simulink model "threelevel_12phase1"  (R2020b)
settings: Solver=FixedStepDiscrete  StartTime=0.0  StopTime=1  FixedStep=Ts_FEA  RelTol=1e-3
model workspace (MAT data in the model file):
  T_10kHz : Simulink.Parameter (value not decoded)
undefined symbols (not defined in the file): Cin, DiscIntNeverNeededParam, ESL, ESR, faif, Jm, kfeed_r, ki_n, kp_n, L, Ld, Line, Lq, ncmd_climb, ncmd_cruise, ncmd_run, ncmd_takeoff, p, Pcmd_climb, Pcmd_cruise, Pcmd_run, Pcmd_takeoff, Rs, Tcmd_run, Tcmd_start, Tcmd_time, time_climb, time_cruise, time_run, time_start, time_takeoff, Ts, Ts_Dead, Ts_FEA, Ts_speedloop, tswitch_climb, tswitch_takeoff, VDC, ws, zero_C1
libraries: powerlib x73, simulink x16, powerlib_meascontrol x16, slpidlib x13
(part 3 of 6)

== matlab function threelevel_12phase1/CurrentLoop/Subsystem/NTSV_7_nearest ==
  data: Alpha input; Beta input; Ta1 output; Ta2 output; Tb1 output; Tb2 output; Tc1 output; Tc2 output; r input; r output
function [Ta1,Ta2,Tb1, Tb2,Tc1,Tc2,r]  = fcn(Alpha,Beta,r)
temp1=Beta;
temp2=0.8660254*Alpha+Beta*0.5;
temp3=temp2-temp1;%0.8660254*Alpha-0.5beta
VecSector1=3;
VecSector2=1;
VecSector3=0;
if temp2>0
    VecSector1=VecSector1-1;
end
if temp3>0
    VecSector1=VecSector1-1;
end
if temp1<0
    VecSector1=7-VecSector1;
end 
switch VecSector1
    case {1,4}  
       if(abs(temp2)>0.5)
           VecSector2=VecSector2+1;
           if(abs(temp3)<0.5)
               VecSector2=VecSector2+1;
               if(abs(temp1)>0.5)
                   VecSector2=VecSector2+1;
               end
           end
       end
       if(temp1<temp3)
           VecSector3=1;
       else
           VecSector3=2;
       end
    case {2,5}
       if(abs(temp1)>0.5)
           VecSector2=VecSector2+1;
           if(abs(temp2)<0.5)
               VecSector2=VecSector2+1;
               if(abs(temp3)>0.5)
                   VecSector2=VecSector2+1;
               end
           end
       end
       if(temp2+temp3>0)
          VecSector3=1;
       else
           VecSector3=2;
       end 
    case {3,6}
       if(abs(temp3)>0.5)
           VecSector2=VecSector2+1;
           if(abs(temp1)<0.5)
               VecSector2=VecSector2+1;
               if(abs(temp2)>0.5)
                   VecSector2=VecSector2+1;
               end
           end
       end
       if(temp1+temp2>0)
          VecSector3=1;
       else
           VecSector3=2;
       end 
    otherwise
        VecSector1=0;
        VecSector2=0;
end
switch VecSector1
    case 1
        switch VecSector2
            case 1
                if(VecSector3==1)
                    Ta1=temp3;
                    Ta2=1;
                    Tb1=0;
                    Tb2=1-temp3;
                    Tc1=0;
                    Tc2=1-temp2-temp1;

                    Tb2=Tb2+Ta1*r;
                    Tc2=Tc2+Ta1*r;
                    Ta1=Ta1+Ta1*r;
                elseif(VecSector3==2)
                    Ta1=temp2+temp3;
                    Ta2=1;
                    Tb1=temp1;
                    Tb2=1;
                    Tc1=0;
                    Tc2=1-temp1;

                    Tc2=Tc2+Tb1*r;
                    Ta1=Ta1+Tb1*r;
                    Tb1=Tb1+Tb1*r;
                else
                    Ta1=temp3;
                    Ta2=1;
                    Tb1=0;
                    Tb2=1-temp3;
                    Tc1=0;
                    Tc2=1-temp2-temp1;

                    Tb2=Tb2+Ta1*r;
                    Tc2=Tc2+Ta1*r;
                    Ta1=Ta1+Ta1*r;
                end
            case 2
                Ta1=temp2;
                Ta2=1;
                Tb1=0;
                Tb2=1-temp3+temp1;
                Tc1=0;
                Tc2=1-temp2;
                
                Ta1=Ta1+Tc2*r;
                Tb2=Tb2+Tc2*r;
                Tc2=Tc2+Tc2*r;
            case 3
                if(VecSector3==1)
                    Ta1=temp2+temp3-0.5;
                    Ta2=1;
                    Tb1=0;
                    Tb2=0.5+temp1;
                    Tc1=0;
                    Tc2=0.5-temp1;

                    Ta1=Ta1+Tc2*r;
                    Tb2=Tb2+Tc2*r;
                    Tc2=Tc2+Tc2*r;
                elseif(VecSector3==2)
                    Ta1=0.5+temp3;
                    Ta2=1;
                    Tb1=0.5-temp3;
                    Tb2=1;
                    Tc1=0;
                    Tc2=1.5-temp1-temp2;

                    Ta1=Ta1+Tb1*r;
                    Tc2=Tc2+Tb1*r;
                    Tb1=Tb1+Tb1*r;
                else
                    Ta1=temp2+temp3-0.5;
                    Ta2=1;
                    Tb1=0;
                    Tb2=0.5+temp1;
                    Tc1=0;
                    Tc2=0.5-temp1;

                    Ta1=Ta1+Tc2*r;
                    Tb2=Tb2+Tc2*r;
                    Tc2=Tc2+Tc2*r;
                end
            case 4
                Ta1=temp2;
                Ta2=1;
                Tb1=temp1-temp3;
                Tb2=1;
                Tc1=0;
                Tc2=1-temp2;

                Ta1=Ta1+Tc2*r;
                Tb1=Tb1+Tc2*r;
                Tc2=Tc2+Tc2*r; 
            otherwise
                Ta1=0;
                Ta2=1;
                Tb1=0;
                Tb2=1;
                Tc1=0;
                Tc2=1;
        end
    case 2
        switch VecSector2
            case 1
                if(VecSector3==1)
                    Ta1=temp2;
                    Ta2=1;
                    Tb1=temp1-temp3;
                    Tb2=1;
                    Tc1=0;
                    Tc2=1-temp2;

                    Tb1=Tb1+Ta1*r;
                    Tc2=Tc2+Ta1*r;
                    Ta1=Ta1+Ta1*r;
                elseif(VecSector3==2)
                    Ta1=0;
                    Ta2=1+temp3;
                    Tb1=-temp3;
                    Tb2=1;
                    Tc1=0;
                    Tc2=1-temp2-temp1;
                    
                    Tc2=Tc2+Tb1*r;
                    Ta2=Ta2+Tb1*r;
                    Tb1=Tb1+Tb1*r;
                else
                    Ta1=temp2;
                    Ta2=1;
                    Tb1=temp1-temp3;
                    Tb2=1;
                    Tc1=0;
                    Tc2=1-temp2;

                    Tb1=Tb1+Ta1*r;
                    Tc2=Tc2+Ta1*r;
                    Ta1=Ta1+Ta1*r;
                end
            case 2
                Ta1=temp2+temp3;
                Ta2=1;
                Tb1=temp1;
                Tb2=1;
                Tc1=0;
                Tc2=1-temp1;
                
                Ta1=Ta1+Tc2*r;
                Tb1=Tb1+Tc2*r;
                Tc2=Tc2+Tc2*r;
            case 3
                if(VecSector3==1)
                    Ta1=0.5+temp3;
                    Ta2=1;
                    Tb1=0.5-temp3;
                    Tb2=1;
                    Tc1=0;
                    Tc2=1.5-temp2-temp1;

                    Tb1=Tb1+Ta1*r;
                    Tc2=Tc2+Ta1*r;
                    Ta1=Ta1+Ta1*r;
                elseif(VecSector3==2)
                    Ta1=0;
                    Ta2=0.5+temp2;
                    Tb1=temp1-temp3-0.5;
                    Tb2=1;
                    Tc1=0;
                    Tc2=0.5-temp2;

                    Tb1=Tb1+Tc2*r;
                    Ta2=Ta2+Tc2*r;
                    Tc2=Tc2+Tc2*r;
                else
                    Ta1=0.5+temp3;
                    Ta2=1;
                    Tb1=0.5-temp3;
                    Tb2=1;
                    Tc1=0;
                    Tc2=1.5-temp2-temp1;

                    Tb1=Tb1+Ta1*r;
                    Tc2=Tc2+Ta1*r;
                    Ta1=Ta1+Ta1*r;
                end
            case 4
                Ta1=0;
                Ta2=1+temp2+temp3;
                Tb1=temp1;
                Tb2=1;
                Tc1=0;
                Tc2=1-temp1;
                
                Ta2=Ta2+Tc2*r;
                Tb1=Tb1+Tc2*r;
                Tc2=Tc2+Tc2*r;
            otherwise
                Ta1=0;
                Ta2=1;
                Tb1=0;
                Tb2=1;
                Tc1=0;
                Tc2=1;
        end
    case 3
        switch VecSector2
            case 1
                if(VecSector3==1)
                    Ta1=0;
                    Ta2=1+temp2+temp3;
                    Tb1=temp1;
                    Tb2=1;
                    Tc1=0;
                    Tc2=1-temp1;

                    Ta2=Ta2+Tb1*r;
                    Tc2=Tc2+Tb1*r;
                    Tb1=Tb1+Tb1*r;
                elseif(VecSector3==2)
                    Ta1=0;
                    Ta2=1+temp2;
                    Tb1=temp1-temp3;
                    Tb2=1;
                    Tc1=-temp2;
                    Tc2=1;

                    Ta2=Ta2+Tc1*r;
                    Tb1=Tb1+Tc1*r;
                    Tc1=Tc1+Tc1*r;
                else
                    Ta1=0;
                    Ta2=1+temp2+temp3;
                    Tb1=temp1;
                    Tb2=1;
                    Tc1=0;
                    Tc2=1-temp1;

                    Ta2=Ta2+Tb1*r;
                    Tc2=Tc2+Tb1*r;
                    Tb1=Tb1+Tb1*r;
                end
            case 2
                Ta1=0;
                Ta2=1+temp3;
                Tb1=-temp3;
                Tb2=1;
                Tc1=0;
                Tc2=1-temp2-temp1;

                Tb1=Tb1+Ta2*r;
                Tc2=Tc2+Ta2*r;
                Ta2=Ta2+Ta2*r;
            case 3
                if(VecSector3==1)
                    Ta1=0;
                    Ta2=0.5+temp2;
                    Tb1=-0.5-temp3+temp1;
                    Tb2=1;
                    Tc1=0;
                    Tc2=0.5-temp2;

                    Tb1=Tb1+Ta2*r;
                    Tc2=Tc2+Ta2*r;
                    Ta2=Ta2+Ta2*r;
                elseif(VecSector3==2)
                    Ta1=0;
                    Ta2=1.5+temp2+temp3;
                    Tb1=0.5+temp1;
                    Tb2=1;
                    Tc1=0.5-temp1;
                    Tc2=1;

                    Tb1=Tb1+Tc1*r;
                    Ta2=Ta2+Tc1*r;
                    Tc1=Tc1+Tc1*r;
                else
                    Ta1=0;
                    Ta2=0.5+temp2;
                    Tb1=-0.5-temp3+temp1;
                    Tb2=1;
                    Tc1=0;
                    Tc2=0.5-temp2;

                    Tb1=Tb1+Ta2*r;
                    Tc2=Tc2+Ta2*r;
                    Ta2=Ta2+Ta2*r; 
                end
            case 4
                Ta1=0;
                Ta2=1+temp3;
                Tb1=-temp3;
                Tb2=1;
                Tc1=-temp2-temp1;
                Tc2=1;
                
                Tb1=Tb1+Ta2*r;
                Tc1=Tc1+Ta2*r;
                Ta2=Ta2+Ta2*r;
            otherwise
                Ta1=0;
                Ta2=1;
                Tb1=0;
                Tb2=1;
                Tc1=0;
                Tc2=1;
        end
    case 4
        switch VecSector2
            case 1
                if(VecSector3==2)
                    Ta1=0;
                    Ta2=1+temp3;
                    Tb1=-temp3;
                    Tb2=1;
                    Tc1=-temp2-temp1;
                    Tc2=1;

                    Ta2=Ta2+Tb1*r;
                    Tc1=Tc1+Tb1*r;
                    Tb1=Tb1+Tb1*r;
                elseif(VecSector3==1)
                    Ta1=0;
                    Ta2=1+temp3+temp2;
                    Tb1=0;
                    Tb2=1+temp1;
                    Tc1=-temp1;
                    Tc2=1;

                    Ta2=Ta2+Tc1*r;
                    Tb2=Tb2+Tc1*r;
                    Tc1=Tc1+Tc1*r;
                else
                    Ta1=0;
                    Ta2=1+temp3;
                    Tb1=-temp3;
                    Tb2=1;
                    Tc1=-temp2-temp1;
                    Tc2=1;

                    Ta2=Ta2+Tb1*r;
                    Tc1=Tc1+Tb1*r;
                    Tb1=Tb1+Tb1*r;
                end
            case 2
                Ta1=0;
                Ta2=1+temp2;
                Tb1=temp1-temp3;
                Tb2=1;
                Tc1=-temp2;
                Tc2=1;
                
                Tb1=Tb1+Ta2*r;
                Tc1=Tc1+Ta2*r;
                Ta2=Ta2+Ta2*r;
            case 3
                if(VecSector3==2)
                    Ta1=0;
                    Ta2=1.5+temp2+temp3;
                    Tb1=0.5+temp1;
                    Tb2=1;
                    Tc1=0.5-temp1;
                    Tc2=1;

                    Ta2=Ta2+Tb1*r;
                    Tc1=Tc1+Tb1*r;
                    Tb1=Tb1+Tb1*r;
                elseif(VecSector3==1)
                    Ta1=0;
                    Ta2=0.5+temp3;
                    Tb1=0;
                    Tb2=0.5-temp3;
                    Tc1=-0.5-temp2-temp1;
                    Tc2=1;

                    Tc1=Tc1+Ta2*r;
                    Tb2=Tb2+Ta2*r;
                    Ta2=Ta2+Ta2*r;
                else
                    Ta1=0;
                    Ta2=1.5+temp2+temp3;
                    Tb1=0.5+temp1;
                    Tb2=1;
                    Tc1=0.5-temp1;
                    Tc2=1;

                    Ta2=Ta2+Tb1*r;
                    Tc1=Tc1+Tb1*r;
                    Tb1=Tb1+Tb1*r;
                end
            case 4
                Ta1=0;
                Ta2=1+temp2;
                Tb1=0;
                Tb2=1+temp1-temp3;
                Tc1=-temp2;
                Tc2=1;
                
                Tc1=Tc1+Ta2*r;
                Tb2=Tb2+Ta2*r;
                Ta2=Ta2+Ta2*r;
            otherwise
                Ta1=0;
                Ta2=1;
                Tb1=0;
                Tb2=1;
                Tc1=0;
                Tc2=1;
        end
    case 5
        switch VecSector2
            case 1
                if(VecSector3==2)
                    Ta1=0;
                    Ta2=1+temp2;
                    Tb1=0;
                    Tb2=1-temp3+temp1;
                    Tc1=-temp2;
                    Tc2=1;

                    Ta2=Ta2+Tc1*r;
                    Tb2=Tb2+Tc1*r;
                    Tc1=Tc1+Tc1*r;
                elseif(VecSector3==1)
                    Ta1=temp3;
                    Ta2=1;
                    Tb1=0;
                    Tb2=1-temp3;
                    Tc1=-temp2-temp1;
                    Tc2=1;

                    Tb2=Tb2+Ta1*r;
                    Tc1=Tc1+Ta1*r;
                    Ta1=Ta1+Ta1*r;
                else
                    Ta1=0;
                    Ta2=1+temp2;
                    Tb1=0;
                    Tb2=1-temp3+temp1;
                    Tc1=-temp2;
                    Tc2=1;

                    Ta2=Ta2+Tc1*r;
                    Tb2=Tb2+Tc1*r;
                    Tc1=Tc1+Tc1*r; 
                end
            case 2
                Ta1=0;
                Ta2=1+temp2+temp3;
                Tb1=0;
                Tb2=1+temp1;
                Tc1=-temp1;
                Tc2=1;
                
                Ta2=Ta2+Tb2*r;
                Tc1=Tc1+Tb2*r;
                Tb2=Tb2+Tb2*r;
            case 3
                if(VecSector3==2)
                    Ta1=0;
                    Ta2=0.5+temp3;
                    Tb1=0;
                    Tb2=0.5-temp3;
                    Tc1=-0.5-temp1-temp2;
                    Tc2=1;

                    Ta2=Ta2+Tb2*r;
                    Tc1=Tc1+Tb2*r;
                    Tb2=Tb2+Tb2*r;
                elseif(VecSector3==1)
                    Ta1=0.5+temp2;
                    Ta2=1;
                    Tb1=0;
                    Tb2=1.5-temp3+temp1;
                    Tc1=0.5-temp2;
                    Tc2=1;
 
                    Tc1=Tc1+Ta1*r;
                    Tb2=Tb2+Ta1*r;
                    Ta1=Ta1+Ta1*r;
                else
                    Ta1=0;
                    Ta2=0.5+temp3;
                    Tb1=0;
                    Tb2=0.5-temp3;
                    Tc1=-0.5-temp1-temp2;
                    Tc2=1;

                    Ta2=Ta2+Tb2*r;
                    Tc1=Tc1+Tb2*r;
                    Tb2=Tb2+Tb2*r;
                end
            case 4
                Ta1=temp2+temp3;
                Ta2=1;
                Tb1=0;
                Tb2=1+temp1;
                Tc1=-temp1;
                Tc2=1;
                
                Ta1=Ta1+Tb2*r;
                Tc1=Tc1+Tb2*r;
                Tb2=Tb2+Tb2*r;
            otherwise
                Ta1=0;
                Ta2=1;
                Tb1=0;
                Tb2=1;
                Tc1=0;
                Tc2=1;
        end
    case 6
        switch VecSector2
            case 1
                if(VecSector3==2)
                    Ta1=temp2+temp3;
                    Ta2=1;
                    Tb1=0;
                    Tb2=1+temp1;
                    Tc1=-temp1;
                    Tc2=1;

                    Ta1=Ta1+Tc1*r;
                    Tb2=Tb2+Tc1*r;
                    Tc1=Tc1+Tc1*r;
                elseif(VecSector3==1)
                    Ta1=temp2;
                    Ta2=1;
                    Tb1=0;
                    Tb2=1+temp1-temp3;
                    Tc1=0;
                    Tc2=1-temp2;

                    Tb2=Tb2+Ta1*r;
                    Tc2=Tc2+Ta1*r;
                    Ta1=Ta1+Ta1*r;
                else
                    Ta1=temp2+temp3;
                    Ta2=1;
                    Tb1=0;
                    Tb2=1+temp1;
                    Tc1=-temp1;
                    Tc2=1;

                    Ta1=Ta1+Tc1*r;
                    Tb2=Tb2+Tc1*r;
                    Tc1=Tc1+Tc1*r;
                end
            case 2
                Ta1=temp3;
                Ta2=1;
                Tb1=0;
                Tb2=1-temp3;
                Tc1=-temp2-temp1;
                Tc2=1;
                
                Ta1=Ta1+Tb2*r;
                Tc1=Tc1+Tb2*r;
                Tb2=Tb2+Tb2*r;
            case 3
                if(VecSector3==2)
                    Ta1=0.5+temp2;
                    Ta2=1;
                    Tb1=0;
                    Tb2=1.5+temp1-temp3;
                    Tc1=0.5-temp2;
                    Tc2=1;

                    Ta1=Ta1+Tc1*r;
                    Tb2=Tb2+Tc1*r;
                    Tc1=Tc1+Tc1*r;
                elseif(VecSector3==1)
                    Ta1=-0.5+temp2+temp3;
                    Ta2=1;
                    Tb1=0;
                    Tb2=0.5+temp1;
                    Tc1=0;
                    Tc2=0.5-temp1;

                    Ta1=Ta1+Tb2*r;
                    Tc2=Tc2+Tb2*r;
                    Tb2=Tb2+Tb2*r;
                else
                    Ta1=0.5+temp2;
                    Ta2=1;
                    Tb1=0;
                    Tb2=1.5+temp1-temp3;
                    Tc1=0.5-temp2;
                    Tc2=1;

                    Ta1=Ta1+Tc1*r;
                    Tb2=Tb2+Tc1*r;
                    Tc1=Tc1+Tc1*r;
                end
            case 4
                Ta1=temp3;
                Ta2=1;
                Tb1=0;
                Tb2=1-temp3;
                Tc1=0;
                Tc2=1-temp2-temp1;
                
                Ta1=Ta1+Tb2*r;
                Tc2=Tc2+Tb2*r;
                Tb2=Tb2+Tb2*r;
            otherwise
                Ta1=0;
                Ta2=1;
                Tb1=0;
                Tb2=1;
                Tc1=0;
                Tc2=1;
        end
    otherwise
        Ta1=0;
        Ta2=1;
        Tb1=0;
        Tb2=1;
        Tc1=0;
        Tc2=1;
end

== matlab function threelevel_12phase1/CurrentLoop/Subsystem2/NTSV_7_nearest ==
  data: Alpha input; Beta input; Ta1 output; Ta2 output; Tb1 output; Tb2 output; Tc1 output; Tc2 output; r input; r output
function [Ta1,Ta2,Tb1, Tb2,Tc1,Tc2,r]  = fcn(Alpha,Beta,r)
temp1=Beta;
temp2=0.8660254*Alpha+Beta*0.5;
temp3=temp2-temp1;%0.8660254*Alpha-0.5beta
VecSector1=3;
VecSector2=1;
VecSector3=0;
if temp2>0
    VecSector1=VecSector1-1;
end
if temp3>0
    VecSector1=VecSector1-1;
end
if temp1<0
    VecSector1=7-VecSector1;
end 
switch VecSector1
    case {1,4}  
       if(abs(temp2)>0.5)
           VecSector2=VecSector2+1;
           if(abs(temp3)<0.5)
               VecSector2=VecSector2+1;
               if(abs(temp1)>0.5)
                   VecSector2=VecSector2+1;
               end
           end
       end
       if(temp1<temp3)
           VecSector3=1;
       else
           VecSector3=2;
       end
    case {2,5}
       if(abs(temp1)>0.5)
           VecSector2=VecSector2+1;
           if(abs(temp2)<0.5)
               VecSector2=VecSector2+1;
               if(abs(temp3)>0.5)
                   VecSector2=VecSector2+1;
               end
           end
       end
       if(temp2+temp3>0)
          VecSector3=1;
       else
           VecSector3=2;
       end 
    case {3,6}
       if(abs(temp3)>0.5)
           VecSector2=VecSector2+1;
           if(abs(temp1)<0.5)
               VecSector2=VecSector2+1;
               if(abs(temp2)>0.5)
                   VecSector2=VecSector2+1;
               end
           end
       end
       if(temp1+temp2>0)
          VecSector3=1;
       else
           VecSector3=2;
       end 
    otherwise
        VecSector1=0;
        VecSector2=0;
end
switch VecSector1
    case 1
        switch VecSector2
            case 1
                if(VecSector3==1)
                    Ta1=temp3;
                    Ta2=1;
                    Tb1=0;
                    Tb2=1-temp3;
                    Tc1=0;
                    Tc2=1-temp2-temp1;

                    Tb2=Tb2+Ta1*r;
                    Tc2=Tc2+Ta1*r;
                    Ta1=Ta1+Ta1*r;
                elseif(VecSector3==2)
                    Ta1=temp2+temp3;
                    Ta2=1;
                    Tb1=temp1;
                    Tb2=1;
                    Tc1=0;
                    Tc2=1-temp1;

                    Tc2=Tc2+Tb1*r;
                    Ta1=Ta1+Tb1*r;
                    Tb1=Tb1+Tb1*r;
                else
                    Ta1=temp3;
                    Ta2=1;
                    Tb1=0;
                    Tb2=1-temp3;
                    Tc1=0;
                    Tc2=1-temp2-temp1;

                    Tb2=Tb2+Ta1*r;
                    Tc2=Tc2+Ta1*r;
                    Ta1=Ta1+Ta1*r;
                end
            case 2
                Ta1=temp2;
                Ta2=1;
                Tb1=0;
                Tb2=1-temp3+temp1;
                Tc1=0;
                Tc2=1-temp2;
                
                Ta1=Ta1+Tc2*r;
                Tb2=Tb2+Tc2*r;
                Tc2=Tc2+Tc2*r;
            case 3
                if(VecSector3==1)
                    Ta1=temp2+temp3-0.5;
                    Ta2=1;
                    Tb1=0;
                    Tb2=0.5+temp1;
                    Tc1=0;
                    Tc2=0.5-temp1;

                    Ta1=Ta1+Tc2*r;
                    Tb2=Tb2+Tc2*r;
                    Tc2=Tc2+Tc2*r;
                elseif(VecSector3==2)
                    Ta1=0.5+temp3;
                    Ta2=1;
                    Tb1=0.5-temp3;
                    Tb2=1;
                    Tc1=0;
                    Tc2=1.5-temp1-temp2;

                    Ta1=Ta1+Tb1*r;
                    Tc2=Tc2+Tb1*r;
                    Tb1=Tb1+Tb1*r;
                else
                    Ta1=temp2+temp3-0.5;
                    Ta2=1;
                    Tb1=0;
                    Tb2=0.5+temp1;
                    Tc1=0;
                    Tc2=0.5-temp1;

                    Ta1=Ta1+Tc2*r;
                    Tb2=Tb2+Tc2*r;
                    Tc2=Tc2+Tc2*r;
                end
            case 4
                Ta1=temp2;
                Ta2=1;
                Tb1=temp1-temp3;
                Tb2=1;
                Tc1=0;
                Tc2=1-temp2;

                Ta1=Ta1+Tc2*r;
                Tb1=Tb1+Tc2*r;
                Tc2=Tc2+Tc2*r; 
            otherwise
                Ta1=0;
                Ta2=1;
                Tb1=0;
                Tb2=1;
                Tc1=0;
                Tc2=1;
        end
    case 2
        switch VecSector2
            case 1
                if(VecSector3==1)
                    Ta1=temp2;
                    Ta2=1;
                    Tb1=temp1-temp3;
                    Tb2=1;
                    Tc1=0;
                    Tc2=1-temp2;

                    Tb1=Tb1+Ta1*r;
                    Tc2=Tc2+Ta1*r;
                    Ta1=Ta1+Ta1*r;
                elseif(VecSector3==2)
                    Ta1=0;
                    Ta2=1+temp3;
                    Tb1=-temp3;
                    Tb2=1;
                    Tc1=0;
                    Tc2=1-temp2-temp1;
                    
                    Tc2=Tc2+Tb1*r;
                    Ta2=Ta2+Tb1*r;
                    Tb1=Tb1+Tb1*r;
                else
                    Ta1=temp2;
                    Ta2=1;
                    Tb1=temp1-temp3;
                    Tb2=1;
                    Tc1=0;
                    Tc2=1-temp2;

                    Tb1=Tb1+Ta1*r;
                    Tc2=Tc2+Ta1*r;
                    Ta1=Ta1+Ta1*r;
                end
            case 2
                Ta1=temp2+temp3;
                Ta2=1;
                Tb1=temp1;
                Tb2=1;
                Tc1=0;
                Tc2=1-temp1;
                
                Ta1=Ta1+Tc2*r;
                Tb1=Tb1+Tc2*r;
                Tc2=Tc2+Tc2*r;
            case 3
                if(VecSector3==1)
                    Ta1=0.5+temp3;
                    Ta2=1;
                    Tb1=0.5-temp3;
                    Tb2=1;
                    Tc1=0;
                    Tc2=1.5-temp2-temp1;

                    Tb1=Tb1+Ta1*r;
                    Tc2=Tc2+Ta1*r;
                    Ta1=Ta1+Ta1*r;
                elseif(VecSector3==2)
                    Ta1=0;
                    Ta2=0.5+temp2;
                    Tb1=temp1-temp3-0.5;
                    Tb2=1;
                    Tc1=0;
                    Tc2=0.5-temp2;

                    Tb1=Tb1+Tc2*r;
                    Ta2=Ta2+Tc2*r;
                    Tc2=Tc2+Tc2*r;
                else
                    Ta1=0.5+temp3;
                    Ta2=1;
                    Tb1=0.5-temp3;
                    Tb2=1;
                    Tc1=0;
                    Tc2=1.5-temp2-temp1;

                    Tb1=Tb1+Ta1*r;
                    Tc2=Tc2+Ta1*r;
                    Ta1=Ta1+Ta1*r;
                end
            case 4
                Ta1=0;
                Ta2=1+temp2+temp3;
                Tb1=temp1;
                Tb2=1;
                Tc1=0;
                Tc2=1-temp1;
                
                Ta2=Ta2+Tc2*r;
                Tb1=Tb1+Tc2*r;
                Tc2=Tc2+Tc2*r;
            otherwise
                Ta1=0;
                Ta2=1;
                Tb1=0;
                Tb2=1;
                Tc1=0;
                Tc2=1;
        end
    case 3
        switch VecSector2
            case 1
                if(VecSector3==1)
                    Ta1=0;
                    Ta2=1+temp2+temp3;
                    Tb1=temp1;
                    Tb2=1;
                    Tc1=0;
                    Tc2=1-temp1;

                    Ta2=Ta2+Tb1*r;
                    Tc2=Tc2+Tb1*r;
                    Tb1=Tb1+Tb1*r;
                elseif(VecSector3==2)
                    Ta1=0;
                    Ta2=1+temp2;
                    Tb1=temp1-temp3;
                    Tb2=1;
                    Tc1=-temp2;
                    Tc2=1;

                    Ta2=Ta2+Tc1*r;
                    Tb1=Tb1+Tc1*r;
                    Tc1=Tc1+Tc1*r;
                else
                    Ta1=0;
                    Ta2=1+temp2+temp3;
                    Tb1=temp1;
                    Tb2=1;
                    Tc1=0;
                    Tc2=1-temp1;

                    Ta2=Ta2+Tb1*r;
                    Tc2=Tc2+Tb1*r;
                    Tb1=Tb1+Tb1*r;
                end
            case 2
                Ta1=0;
                Ta2=1+temp3;
                Tb1=-temp3;
                Tb2=1;
                Tc1=0;
                Tc2=1-temp2-temp1;

                Tb1=Tb1+Ta2*r;
                Tc2=Tc2+Ta2*r;
                Ta2=Ta2+Ta2*r;
            case 3
                if(VecSector3==1)
                    Ta1=0;
                    Ta2=0.5+temp2;
                    Tb1=-0.5-temp3+temp1;
                    Tb2=1;
                    Tc1=0;
                    Tc2=0.5-temp2;

                    Tb1=Tb1+Ta2*r;
                    Tc2=Tc2+Ta2*r;
                    Ta2=Ta2+Ta2*r;
                elseif(VecSector3==2)
                    Ta1=0;
                    Ta2=1.5+temp2+temp3;
                    Tb1=0.5+temp1;
                    Tb2=1;
                    Tc1=0.5-temp1;
                    Tc2=1;

                    Tb1=Tb1+Tc1*r;
                    Ta2=Ta2+Tc1*r;
                    Tc1=Tc1+Tc1*r;
                else
                    Ta1=0;
                    Ta2=0.5+temp2;
                    Tb1=-0.5-temp3+temp1;
                    Tb2=1;
                    Tc1=0;
                    Tc2=0.5-temp2;

                    Tb1=Tb1+Ta2*r;
                    Tc2=Tc2+Ta2*r;
                    Ta2=Ta2+Ta2*r; 
                end
            case 4
                Ta1=0;
                Ta2=1+temp3;
                Tb1=-temp3;
                Tb2=1;
                Tc1=-temp2-temp1;
                Tc2=1;
                
                Tb1=Tb1+Ta2*r;
                Tc1=Tc1+Ta2*r;
                Ta2=Ta2+Ta2*r;
            otherwise
                Ta1=0;
                Ta2=1;
                Tb1=0;
                Tb2=1;
                Tc1=0;
                Tc2=1;
        end
    case 4
        switch VecSector2
            case 1
                if(VecSector3==2)
                    Ta1=0;
                    Ta2=1+temp3;
                    Tb1=-temp3;
                    Tb2=1;
                    Tc1=-temp2-temp1;
                    Tc2=1;

                    Ta2=Ta2+Tb1*r;
                    Tc1=Tc1+Tb1*r;
                    Tb1=Tb1+Tb1*r;
                elseif(VecSector3==1)
                    Ta1=0;
                    Ta2=1+temp3+temp2;
                    Tb1=0;
                    Tb2=1+temp1;
                    Tc1=-temp1;
                    Tc2=1;

                    Ta2=Ta2+Tc1*r;
                    Tb2=Tb2+Tc1*r;
                    Tc1=Tc1+Tc1*r;
                else
                    Ta1=0;
                    Ta2=1+temp3;
                    Tb1=-temp3;
                    Tb2=1;
                    Tc1=-temp2-temp1;
                    Tc2=1;

                    Ta2=Ta2+Tb1*r;
                    Tc1=Tc1+Tb1*r;
                    Tb1=Tb1+Tb1*r;
                end
            case 2
                Ta1=0;
                Ta2=1+temp2;
                Tb1=temp1-temp3;
                Tb2=1;
                Tc1=-temp2;
                Tc2=1;
                
                Tb1=Tb1+Ta2*r;
                Tc1=Tc1+Ta2*r;
                Ta2=Ta2+Ta2*r;
            case 3
                if(VecSector3==2)
                    Ta1=0;
                    Ta2=1.5+temp2+temp3;
                    Tb1=0.5+temp1;
                    Tb2=1;
                    Tc1=0.5-temp1;
                    Tc2=1;

                    Ta2=Ta2+Tb1*r;
                    Tc1=Tc1+Tb1*r;
                    Tb1=Tb1+Tb1*r;
                elseif(VecSector3==1)
                    Ta1=0;
                    Ta2=0.5+temp3;
                    Tb1=0;
                    Tb2=0.5-temp3;
                    Tc1=-0.5-temp2-temp1;
                    Tc2=1;

                    Tc1=Tc1+Ta2*r;
                    Tb2=Tb2+Ta2*r;
                    Ta2=Ta2+Ta2*r;
                else
                    Ta1=0;
                    Ta2=1.5+temp2+temp3;
                    Tb1=0.5+temp1;
                    Tb2=1;
                    Tc1=0.5-temp1;
                    Tc2=1;

                    Ta2=Ta2+Tb1*r;
                    Tc1=Tc1+Tb1*r;
                    Tb1=Tb1+Tb1*r;
                end
            case 4
                Ta1=0;
                Ta2=1+temp2;
                Tb1=0;
                Tb2=1+temp1-temp3;
                Tc1=-temp2;
                Tc2=1;
                
                Tc1=Tc1+Ta2*r;
                Tb2=Tb2+Ta2*r;
                Ta2=Ta2+Ta2*r;
            otherwise
                Ta1=0;
                Ta2=1;
                Tb1=0;
                Tb2=1;
                Tc1=0;
                Tc2=1;
        end
    case 5
        switch VecSector2
            case 1
                if(VecSector3==2)
                    Ta1=0;
                    Ta2=1+temp2;
                    Tb1=0;
                    Tb2=1-temp3+temp1;
                    Tc1=-temp2;
                    Tc2=1;

                    Ta2=Ta2+Tc1*r;
                    Tb2=Tb2+Tc1*r;
                    Tc1=Tc1+Tc1*r;
                elseif(VecSector3==1)
                    Ta1=temp3;
                    Ta2=1;
                    Tb1=0;
                    Tb2=1-temp3;
                    Tc1=-temp2-temp1;
                    Tc2=1;

                    Tb2=Tb2+Ta1*r;
                    Tc1=Tc1+Ta1*r;
                    Ta1=Ta1+Ta1*r;
                else
                    Ta1=0;
                    Ta2=1+temp2;
                    Tb1=0;
                    Tb2=1-temp3+temp1;
                    Tc1=-temp2;
                    Tc2=1;

                    Ta2=Ta2+Tc1*r;
                    Tb2=Tb2+Tc1*r;
                    Tc1=Tc1+Tc1*r; 
                end
            case 2
                Ta1=0;
                Ta2=1+temp2+temp3;
                Tb1=0;
                Tb2=1+temp1;
                Tc1=-temp1;
                Tc2=1;
                
                Ta2=Ta2+Tb2*r;
                Tc1=Tc1+Tb2*r;
                Tb2=Tb2+Tb2*r;
            case 3
                if(VecSector3==2)
                    Ta1=0;
                    Ta2=0.5+temp3;
                    Tb1=0;
                    Tb2=0.5-temp3;
                    Tc1=-0.5-temp1-temp2;
                    Tc2=1;

                    Ta2=Ta2+Tb2*r;
                    Tc1=Tc1+Tb2*r;
                    Tb2=Tb2+Tb2*r;
                elseif(VecSector3==1)
                    Ta1=0.5+temp2;
                    Ta2=1;
                    Tb1=0;
                    Tb2=1.5-temp3+temp1;
                    Tc1=0.5-temp2;
                    Tc2=1;
 
                    Tc1=Tc1+Ta1*r;
                    Tb2=Tb2+Ta1*r;
                    Ta1=Ta1+Ta1*r;
                else
                    Ta1=0;
                    Ta2=0.5+temp3;
                    Tb1=0;
                    Tb2=0.5-temp3;
                    Tc1=-0.5-temp1-temp2;
                    Tc2=1;

                    Ta2=Ta2+Tb2*r;
                    Tc1=Tc1+Tb2*r;
                    Tb2=Tb2+Tb2*r;
                end
            case 4
                Ta1=temp2+temp3;
                Ta2=1;
                Tb1=0;
                Tb2=1+temp1;
                Tc1=-temp1;
                Tc2=1;
                
                Ta1=Ta1+Tb2*r;
                Tc1=Tc1+Tb2*r;
                Tb2=Tb2+Tb2*r;
            otherwise
                Ta1=0;
                Ta2=1;
                Tb1=0;
                Tb2=1;
                Tc1=0;
                Tc2=1;
        end
    case 6
        switch VecSector2
            case 1
                if(VecSector3==2)
                    Ta1=temp2+temp3;
                    Ta2=1;
                    Tb1=0;
                    Tb2=1+temp1;
                    Tc1=-temp1;
                    Tc2=1;

                    Ta1=Ta1+Tc1*r;
                    Tb2=Tb2+Tc1*r;
                    Tc1=Tc1+Tc1*r;
                elseif(VecSector3==1)
                    Ta1=temp2;
                    Ta2=1;
                    Tb1=0;
                    Tb2=1+temp1-temp3;
                    Tc1=0;
                    Tc2=1-temp2;

                    Tb2=Tb2+Ta1*r;
                    Tc2=Tc2+Ta1*r;
                    Ta1=Ta1+Ta1*r;
                else
                    Ta1=temp2+temp3;
                    Ta2=1;
                    Tb1=0;
                    Tb2=1+temp1;
                    Tc1=-temp1;
                    Tc2=1;

                    Ta1=Ta1+Tc1*r;
                    Tb2=Tb2+Tc1*r;
                    Tc1=Tc1+Tc1*r;
                end
            case 2
                Ta1=temp3;
                Ta2=1;
                Tb1=0;
                Tb2=1-temp3;
                Tc1=-temp2-temp1;
                Tc2=1;
                
                Ta1=Ta1+Tb2*r;
                Tc1=Tc1+Tb2*r;
                Tb2=Tb2+Tb2*r;
            case 3
                if(VecSector3==2)
                    Ta1=0.5+temp2;
                    Ta2=1;
                    Tb1=0;
                    Tb2=1.5+temp1-temp3;
                    Tc1=0.5-temp2;
                    Tc2=1;

                    Ta1=Ta1+Tc1*r;
                    Tb2=Tb2+Tc1*r;
                    Tc1=Tc1+Tc1*r;
                elseif(VecSector3==1)
                    Ta1=-0.5+temp2+temp3;
                    Ta2=1;
                    Tb1=0;
                    Tb2=0.5+temp1;
                    Tc1=0;
                    Tc2=0.5-temp1;

                    Ta1=Ta1+Tb2*r;
                    Tc2=Tc2+Tb2*r;
                    Tb2=Tb2+Tb2*r;
                else
                    Ta1=0.5+temp2;
                    Ta2=1;
                    Tb1=0;
                    Tb2=1.5+temp1-temp3;
                    Tc1=0.5-temp2;
                    Tc2=1;

                    Ta1=Ta1+Tc1*r;
                    Tb2=Tb2+Tc1*r;
                    Tc1=Tc1+Tc1*r;
                end
            case 4
                Ta1=temp3;
                Ta2=1;
                Tb1=0;
                Tb2=1-temp3;
                Tc1=0;
                Tc2=1-temp2-temp1;
                
                Ta1=Ta1+Tb2*r;
                Tc2=Tc2+Tb2*r;
                Tb2=Tb2+Tb2*r;
            otherwise
                Ta1=0;
                Ta2=1;
                Tb1=0;
                Tb2=1;
                Tc1=0;
                Tc2=1;
        end
    otherwise
        Ta1=0;
        Ta2=1;
        Tb1=0;
        Tb2=1;
        Tc1=0;
        Tc2=1;
end

== matlab function threelevel_12phase1/CurrentLoop/NTSV_7_normol ==
  data: Alpha input; Beta input; Ta1 output; Ta2 output; Tb1 output; Tb2 output; Tc1 output; Tc2 output; r input; VecSector1 output
function [Ta1,Ta2,Tb1,Tb2,Tc1,Tc2,VecSector1]  = fcn(Alpha,Beta,r)
temp1=Beta;
temp2=0.8660254*Alpha+Beta*0.5;
temp3=temp2-temp1;%0.8660254*Alpha-0.5beta
VecSector1=3;
VecSector2=1;

if temp2>0
    VecSector1=VecSector1-1;
end
if temp3>0
    VecSector1=VecSector1-1;
end
if temp1<0
    VecSector1=7-VecSector1;
end 
switch VecSector1
    case {1,4}  
       if(abs(temp2)>0.5)
           VecSector2=VecSector2+1;
           if(abs(temp3)<0.5)
               VecSector2=VecSector2+1;
               if(abs(temp1)>0.5)
                   VecSector2=VecSector2+1;
               end
           end
       end
    case {2,5}
       if(abs(temp1)>0.5)
           VecSector2=VecSector2+1;
           if(abs(temp2)<0.5)
               VecSector2=VecSector2+1;
               if(abs(temp3)>0.5)
                   VecSector2=VecSector2+1;
               end
           end
       end
    case {3,6}
       if(abs(temp3)>0.5)
           VecSector2=VecSector2+1;
           if(abs(temp1)<0.5)
               VecSector2=VecSector2+1;
               if(abs(temp2)>0.5)
                   VecSector2=VecSector2+1;
               end
           end
       end
    otherwise
        VecSector1=0;
        VecSector2=0;
end

switch VecSector1
    case 1
        switch VecSector2
            case 1
                Ta1=temp3;
                Ta2=1;
                Tb1=0;
                Tb2=1-temp3;
                Tc1=0;
                Tc2=1-temp2-temp1;

                Tb2=Tb2+Ta1*r;
                Tc2=Tc2+Ta1*r;
                Ta1=Ta1+Ta1*r;
            case 2
                Ta1=temp2;
                Ta2=1;
                Tb1=0;
                Tb2=1-temp3+temp1;
                Tc1=0;
                Tc2=1-temp2;
                
                Ta1=Ta1+Tc2*r;
                Tb2=Tb2+Tc2*r;
                Tc2=Tc2+Tc2*r;
            case 3
                Ta1=temp2+temp3-0.5;
                Ta2=1;
                Tb1=0;
                Tb2=0.5+temp1;
                Tc1=0;
                Tc2=0.5-temp1;

                Ta1=Ta1+Tc2*r;
                Tb2=Tb2+Tc2*r;
                Tc2=Tc2+Tc2*r;
            case 4
                Ta1=temp2;
                Ta2=1;
                Tb1=temp1-temp3;
                Tb2=1;
                Tc1=0;
                Tc2=1-temp2;

                Ta1=Ta1+Tc2*r;
                Tb1=Tb1+Tc2*r;
                Tc2=Tc2+Tc2*r; 
            otherwise
                Ta1=0;
                Ta2=1;
                Tb1=0;
                Tb2=1;
                Tc1=0;
                Tc2=1;
        end
    case 2
        switch VecSector2
            case 1
                Ta1=temp2;
                Ta2=1;
                Tb1=temp1-temp3;
                Tb2=1;
                Tc1=0;
                Tc2=1-temp2;

                Tb1=Tb1+Ta1*r;
                Tc2=Tc2+Ta1*r;
                Ta1=Ta1+Ta1*r;
            case 2
                Ta1=temp2+temp3;
                Ta2=1;
                Tb1=temp1;
                Tb2=1;
                Tc1=0;
                Tc2=1-temp1;
                
                Ta1=Ta1+Tc2*r;
                Tb1=Tb1+Tc2*r;
                Tc2=Tc2+Tc2*r;
            case 3
                Ta1=0.5+temp3;
                Ta2=1;
                Tb1=0.5-temp3;
                Tb2=1;
                Tc1=0;
                Tc2=1.5-temp2-temp1;

                Tb1=Tb1+Ta1*r;
                Tc2=Tc2+Ta1*r;
                Ta1=Ta1+Ta1*r;
            case 4
                Ta1=0;
                Ta2=1+temp2+temp3;
                Tb1=temp1;
                Tb2=1;
                Tc1=0;
                Tc2=1-temp1;
                
                Ta2=Ta2+Tc2*r;
                Tb1=Tb1+Tc2*r;
                Tc2=Tc2+Tc2*r;
            otherwise
                Ta1=0;
                Ta2=1;
                Tb1=0;
                Tb2=1;
                Tc1=0;
                Tc2=1;
        end
    case 3
        switch VecSector2
            case 1
                Ta1=0;
                Ta2=1+temp2+temp3;
                Tb1=temp1;
                Tb2=1;
                Tc1=0;
                Tc2=1-temp1;

                Ta2=Ta2+Tb1*r;
                Tc2=Tc2+Tb1*r;
                Tb1=Tb1+Tb1*r;
            case 2
                Ta1=0;
                Ta2=1+temp3;
                Tb1=-temp3;
                Tb2=1;
                Tc1=0;
                Tc2=1-temp2-temp1;

                Tb1=Tb1+Ta2*r;
                Tc2=Tc2+Ta2*r;
                Ta2=Ta2+Ta2*r;
            case 3
                Ta1=0;
                Ta2=0.5+temp2;
                Tb1=-0.5-temp3+temp1;
                Tb2=1;
                Tc1=0;
                Tc2=0.5-temp2;

                Tb1=Tb1+Ta2*r;
                Tc2=Tc2+Ta2*r;
                Ta2=Ta2+Ta2*r;
            case 4
                Ta1=0;
                Ta2=1+temp3;
                Tb1=-temp3;
                Tb2=1;
                Tc1=-temp2-temp1;
                Tc2=1;
                
                Tb1=Tb1+Ta2*r;
                Tc1=Tc1+Ta2*r;
                Ta2=Ta2+Ta2*r;
            otherwise
                Ta1=0;
                Ta2=1;
                Tb1=0;
                Tb2=1;
                Tc1=0;
                Tc2=1;
        end
    case 4
        switch VecSector2
            case 1
                Ta1=0;
                Ta2=1+temp3;
                Tb1=-temp3;
                Tb2=1;
                Tc1=-temp2-temp1;
                Tc2=1;

                Ta2=Ta2+Tb1*r;
                Tc1=Tc1+Tb1*r;
                Tb1=Tb1+Tb1*r;
            case 2
                Ta1=0;
                Ta2=1+temp2;
                Tb1=temp1-temp3;
                Tb2=1;
                Tc1=-temp2;
                Tc2=1;
                
                Tb1=Tb1+Ta2*r;
                Tc1=Tc1+Ta2*r;
                Ta2=Ta2+Ta2*r;
            case 3
                Ta1=0;
                Ta2=1.5+temp2+temp3;
                Tb1=0.5+temp1;
                Tb2=1;
                Tc1=0.5-temp1;
                Tc2=1;

                Ta2=Ta2+Tb1*r;
                Tc1=Tc1+Tb1*r;
                Tb1=Tb1+Tb1*r;
            case 4
                Ta1=0;
                Ta2=1+temp2;
                Tb1=0;
                Tb2=1+temp1-temp3;
                Tc1=-temp2;
                Tc2=1;
                
                Ta2=Ta2+Tb2*r;
                Tc1=Tc1+Tb2*r;
                Tb2=Tb2+Tb2*r;
            otherwise
                Ta1=0;
                Ta2=1;
                Tb1=0;
                Tb2=1;
                Tc1=0;
                Tc2=1;
        end
    case 5
        switch VecSector2
            case 1
                Ta1=0;
                Ta2=1+temp2;
                Tb1=0;
                Tb2=1-temp3+temp1;
                Tc1=-temp2;
                Tc2=1;

                Ta2=Ta2+Tc1*r;
                Tb2=Tb2+Tc1*r;
                Tc1=Tc1+Tc1*r;
            case 2
                Ta1=0;
                Ta2=1+temp2+temp3;
                Tb1=0;
                Tb2=1+temp1;
                Tc1=-temp1;
                Tc2=1;
                
                Ta2=Ta2+Tb2*r;
                Tc1=Tc1+Tb2*r;
                Tb2=Tb2+Tb2*r;
            case 3
                Ta1=0;
                Ta2=0.5+temp3;
                Tb1=0;
                Tb2=0.5-temp3;
                Tc1=-0.5-temp1-temp2;
                Tc2=1;

                Ta2=Ta2+Tb2*r;
                Tc1=Tc1+Tb2*r;
                Tb2=Tb2+Tb2*r;
            case 4
                Ta1=temp2+temp3;
                Ta2=1;
                Tb1=0;
                Tb2=1+temp1;
                Tc1=-temp1;
                Tc2=1;
                
                Ta1=Ta1+Tb2*r;
                Tc1=Tc1+Tb2*r;
                Tb2=Tb2+Tb2*r;
            otherwise
                Ta1=0;
                Ta2=1;
                Tb1=0;
                Tb2=1;
                Tc1=0;
                Tc2=1;
        end
    case 6
        switch VecSector2
            case 1
                Ta1=temp2+temp3;
                Ta2=1;
                Tb1=0;
                Tb2=1+temp1;
                Tc1=-temp1;
                Tc2=1;

                Ta1=Ta1+Tc1*r;
                Tb2=Tb2+Tc1*r;
                Tc1=Tc1+Tc1*r;
            case 2
                Ta1=temp3;
                Ta2=1;
                Tb1=0;
                Tb2=1-temp3;
                Tc1=-temp2-temp1;
                Tc2=1;
                
                Ta1=Ta1+Tb2*r;
                Tc1=Tc1+Tb2*r;
                Tb2=Tb2+Tb2*r;
            case 3
                Ta1=0.5+temp2;
                Ta2=1;
                Tb1=0;
                Tb2=1.5+temp1-temp3;
                Tc1=0.5-temp2;
                Tc2=1;

                Ta1=Ta1+Tc1*r;
                Tb2=Tb2+Tc1*r;
                Tc1=Tc1+Tc1*r;
            case 4
                Ta1=temp3;
                Ta2=1;
                Tb1=0;
                Tb2=1-temp3;
                Tc1=0;
                Tc2=1-temp2-temp1;
                
                Ta1=Ta1+Tb2*r;
                Tc2=Tc2+Tb2*r;
                Tb2=Tb2+Tb2*r;
            otherwise
                Ta1=0;
                Ta2=1;
                Tb1=0;
                Tb2=1;
                Tc1=0;
                Tc2=1;
        end
    otherwise
        Ta1=0;
        Ta2=1;
        Tb1=0;
        Tb2=1;
        Tc1=0;
        Tc2=1;
end

== matlab function threelevel_12phase1/CurrentLoop/VSPWM ==
  data: Alpha input; Ta1 output; Beta input; Ta2 output; Tb1 output; Tb2 output; Tc1 output; Tc2 output; r input; VecSector1 output
function [Ta1,Ta2,Tb1,Tb2,Tc1,Tc2,VecSector1] = VSVPWM(Alpha,Beta,r)

temp1=Beta;
temp2=0.8660254*Alpha+Beta*0.5;
temp3=temp2-temp1;%0.8660254*Alpha-0.5beta
VecSector1=3;

if temp2>0
    VecSector1=VecSector1-1;
end
if temp3>0
    VecSector1=VecSector1-1;
end
if temp1<0
    VecSector1=7-VecSector1;
end 

switch VecSector1
    case 1
       Ta1=temp2;
       Ta2=1;
       Tb1=temp1;
       Tb2=1-temp3;
       Tc1=0;
       Tc2=1-temp2;
       
       Ta1=Ta1+temp2*r;
       Tc2=Tc2+temp2*r;
    case 2
       Ta1=temp2;
       Ta2=1+temp3;
       Tb1=temp1;
       Tb2=1;
       Tc1=0;
       Tc2=1-temp1;
       
       Tb1=Tb1+temp1*r;
       Tc2=Tc2+temp1*r;
    case 3
       Ta1=0;
       Ta2=1+temp3;
       Tb1=-temp3;
       Tb2=1;
       Tc1=-temp2;
       Tc2=1-temp1;
       
       Ta2=Ta2-temp3*r;
       Tb1=Tb1-temp3*r;
    case 4
       Ta1=0;
       Ta2=1+temp2;
       Tb1=-temp3;
       Tb2=1+temp1;
       Tc1=-temp2;
       Tc2=1;
       
       Ta2=Ta2-temp2*r;
       Tc1=Tc1-temp2*r;
    case 5
       Ta1=temp3;
       Ta2=1+temp2;
       Tb1=0;
       Tb2=1+temp1;
       Tc1=-temp1;
       Tc2=1;
       
       Tb2=Tb2-temp1*r;
       Tc1=Tc1-temp1*r;
    case 6
       Ta1=temp3;
       Ta2=1;
       Tb1=0;
       Tb2=1-temp3;
       Tc1=-temp1;
       Tc2=1-temp2;
       
       Ta1=Ta1+temp3*r;
       Tb2=Tb2+temp3*r;
    otherwise
       Ta1=0;
       Ta2=1;
       Tb1=0;
       Tb2=1;
       Tc1=0;
       Tc2=1; 
end
end
